simulink model "dron_filtro_complementario_version2015_Orientacion2"  (R2015b)
settings: Solver=FixedStepDiscrete  StartTime=0.0  StopTime=inf  FixedStep=0.03  RelTol=1e-3
undefined symbols (not defined in the file): DiscIntNeverNeededParam
libraries: simulink x5, arduinolib x4, RASPlib x2
settings Model: SimulationMode=external  ExtModeTrigDuration=2  Creator=jorge  LastModifiedBy=jorge
settings OptimizationCC: OptimizeModelRefInitCode=on  LifeSpan=Inf  MaxStackSize=64
settings HardwareCC: ProdBitPerInt=16  ProdBitPerPointer=16  ProdLargestAtomicFloat=None  ProdWordSize=8  ProdHWDeviceType=Atmel->AVR
settings RTWCC: SystemTargetFile=ert.tlc  TemplateMakefile=ert_default_tmf  Description=Embedded Coder  Toolchain=Arduino AVR v1.6.1  BuildConfiguration=Faster Runs
settings CodeAppCC: IgnoreCustomStorageClasses=off
settings ERTTargetCC: SupportContinuousTime=on  SupportVariableSizeSignals=on  ExtMode=on  ExtModeMexFile=ext_serial_win32_comm_rtt  ExtModeMexArgs=0 5 115200

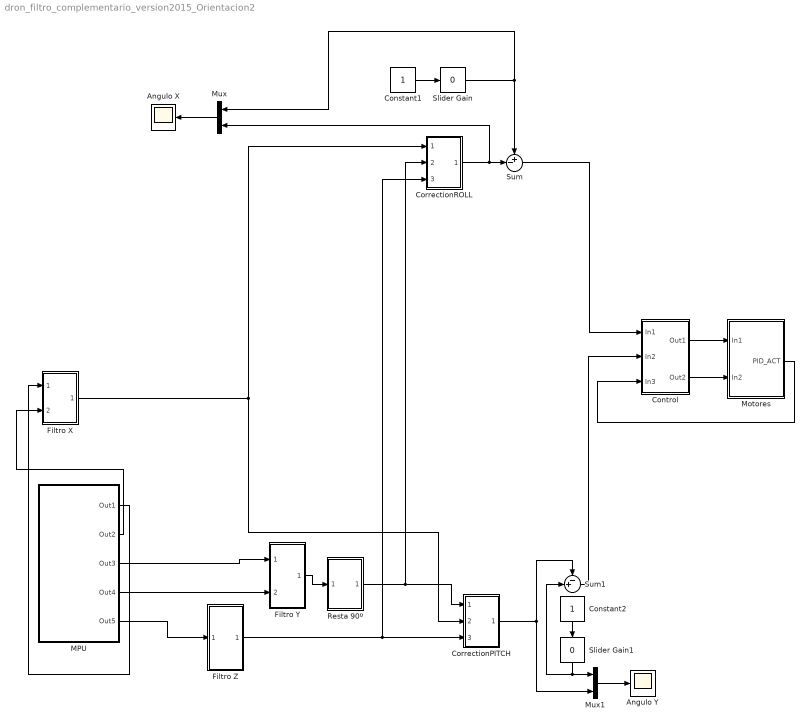
== system dron_filtro_complementario_version2015_Orientacion2 ==
  Angulo X : Scope
  Angulo Y : Scope
  Constant1 : Constant
  Constant2 : Constant
  Control : Subsystem
  CorrectionPITCH : Subsystem
  CorrectionROLL : Subsystem
  Filtro X : Subsystem
  Filtro Y : Subsystem
  "Filtro Z " : Subsystem
  "MPU " : Subsystem
  "Motores " : Subsystem
  Mux : Mux  Inputs=2
  Mux1 : Mux  Inputs=2
  Resta 90º : Subsystem
  Slider Gain : simulink/Math Operations/Slider Gain  low=-25  gain=0  high=35
  Slider Gain1 : simulink/Math Operations/Slider Gain  low=-25  gain=0  high=35
  Sum : Sum  Inputs=+-|
  Sum1 : Sum  Inputs=-+|
  wires:
  "MPU "/1(Out1) -> Filtro X/1(In1)
  "MPU "/2(Out2) -> Filtro X/2(In2)
  Mux/1 -> Angulo X/1
  Constant1/1 -> Slider Gain/1
  Slider Gain/1 -> Sum/1, Mux/1
  "MPU "/3(Out3) -> Filtro Y/1(In1)
  "MPU "/4(Out4) -> Filtro Y/2(In2)
  Constant2/1 -> Slider Gain1/1
  Mux1/1 -> Angulo Y/1
  "MPU "/5(Out5) -> "Filtro Z "/1(In1)
  Filtro X/1(Out3) -> CorrectionPITCH/2(In2), CorrectionROLL/1(In1)
  Slider Gain1/1 -> Mux1/1, Sum1/2
  Filtro Y/1(Out3) -> Resta 90º/1(In1)
  Resta 90º/1(Out1) -> CorrectionPITCH/1(In1), CorrectionROLL/2(In2)
  "Filtro Z "/1(Out3) -> CorrectionROLL/3(In3), CorrectionPITCH/3(In3)
  CorrectionPITCH/1(Out1) -> Sum1/1, Mux1/2
  CorrectionROLL/1(Out1) -> Sum/2, Mux/2
  Sum/1 -> Control/1(In1)
  Sum1/1 -> Control/2(In2)
  Control/1(Out1) -> "Motores "/1(In1)
  Control/2(Out2) -> "Motores "/2(In2)
  "Motores "/1("PID_ACT ") -> Control/3(In3)

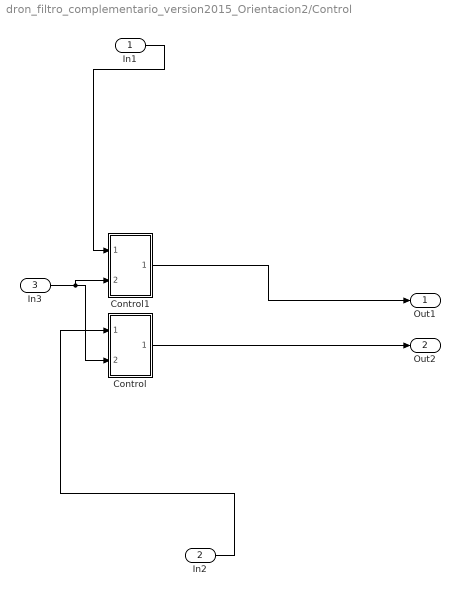
== system dron_filtro_complementario_version2015_Orientacion2/Control ==
  In1 : Inport
  In2 : Inport  Port=2
  In3 : Inport  Port=3
  Control : Subsystem
  Control1 : Subsystem
  Out1 : Outport
  Out2 : Outport  Port=2
  wires:
  Control1/1(Out1) -> Out1/1
  Control/1(Out1) -> Out2/1
  In2/1 -> Control/1(In1)
  In1/1 -> Control1/1(In1)
  In3/1 -> Control/2(Threshold), Control1/2(Threshold)

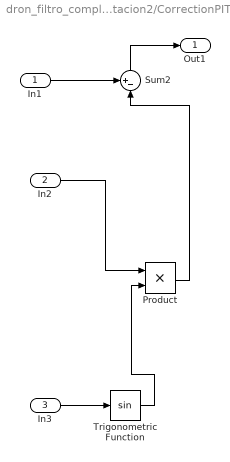
== system dron_filtro_complementario_version2015_Orientacion2/CorrectionPITCH ==
  In1 : Inport
  In2 : Inport  Port=2
  In3 : Inport  Port=3
  Product : Product
  Sum2 : Sum  Inputs=+-|
  Trigonometric Function : Trigonometry
  Out1 : Outport
  wires:
  Trigonometric Function/1 -> Product/2
  Product/1 -> Sum2/2
  In1/1 -> Sum2/1
  In3/1 -> Trigonometric Function/1
  Sum2/1 -> Out1/1
  In2/1 -> Product/1

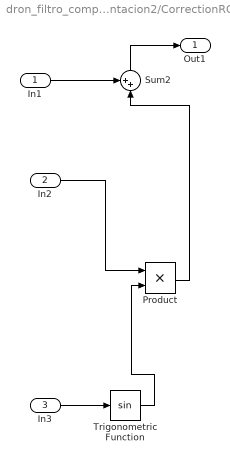
== system dron_filtro_complementario_version2015_Orientacion2/CorrectionROLL ==
  In1 : Inport
  In2 : Inport  Port=2
  In3 : Inport  Port=3
  Product : Product
  Sum2 : Sum  Inputs=++|
  Trigonometric Function : Trigonometry
  Out1 : Outport
  wires:
  Trigonometric Function/1 -> Product/2
  Product/1 -> Sum2/2
  In1/1 -> Sum2/1
  In3/1 -> Trigonometric Function/1
  Sum2/1 -> Out1/1
  In2/1 -> Product/1

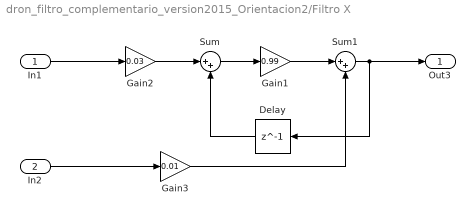
== system dron_filtro_complementario_version2015_Orientacion2/Filtro X ==
  In1 : Inport
  In2 : Inport  Port=2
  Delay : Delay  DelayLength=1  InitialCondition=0
  Gain1 : Gain  Gain=0.99
  Gain2 : Gain  Gain=0.03
  Gain3 : Gain  Gain=0.01
  Sum : Sum  Inputs=|++
  Sum1 : Sum  Inputs=|++
  Out3 : Outport
  wires:
  Delay/1 -> Sum/2
  Sum/1 -> Gain1/1
  In2/1 -> Gain3/1
  Gain1/1 -> Sum1/1
  Sum1/1 -> Out3/1, Delay/1
  In1/1 -> Gain2/1
  Gain2/1 -> Sum/1
  Gain3/1 -> Sum1/2

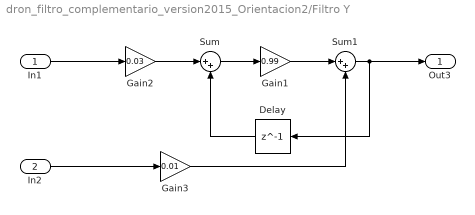
== system dron_filtro_complementario_version2015_Orientacion2/Filtro Y ==
  In1 : Inport
  In2 : Inport  Port=2
  Delay : Delay  DelayLength=1  InitialCondition=0
  Gain1 : Gain  Gain=0.99
  Gain2 : Gain  Gain=0.03
  Gain3 : Gain  Gain=0.01
  Sum : Sum  Inputs=|++
  Sum1 : Sum  Inputs=|++
  Out3 : Outport
  wires:
  Delay/1 -> Sum/2
  Sum/1 -> Gain1/1
  In2/1 -> Gain3/1
  Gain1/1 -> Sum1/1
  Sum1/1 -> Out3/1, Delay/1
  In1/1 -> Gain2/1
  Gain2/1 -> Sum/1
  Gain3/1 -> Sum1/2

== system dron_filtro_complementario_version2015_Orientacion2/Filtro Z  ==
  In1 : Inport
  Discrete-Time Integrator : DiscreteIntegrator  InitialConditionSetting=State (most efficient)  SampleTime=-1  ICPrevOutput=DiscIntNeverNeededParam  ICPrevScaledInput=DiscIntNeverNeededParam
  Gain : Gain  Gain=3.1416/180
  Out3 : Outport
  wires:
  In1/1 -> Discrete-Time Integrator/1
  Gain/1 -> Out3/1
  Discrete-Time Integrator/1 -> Gain/1

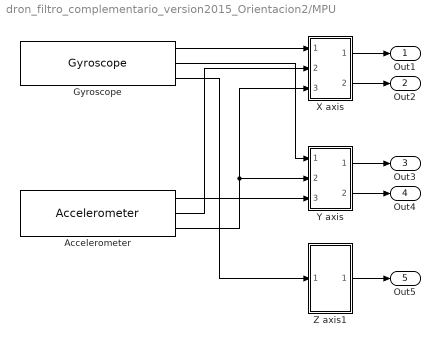
== system dron_filtro_complementario_version2015_Orientacion2/MPU  ==
  Accelerometer : RASPlib/Accelerometer  SimulateUsing=Code generation
  Gyroscope : RASPlib/Gyroscope  DLPFmode=0
  X axis : Subsystem
  Y axis : Subsystem
  Z axis1 : Subsystem
  Out1 : Outport
  Out2 : Outport  Port=2
  Out3 : Outport  Port=3
  Out4 : Outport  Port=4
  Out5 : Outport  Port=5
  wires:
  Gyroscope/3 -> Z axis1/1(In1)
  Gyroscope/1 -> X axis/1(In1)
  Accelerometer/2 -> X axis/2(In2)
  Accelerometer/3 -> Y axis/2(In2), X axis/3(In3)
  X axis/1(Out1) -> Out1/1
  X axis/2(Out2) -> Out2/1
  Gyroscope/2 -> Y axis/1(In1)
  Y axis/1(Out1) -> Out3/1
  Y axis/2(Out2) -> Out4/1
  Z axis1/1(Out1) -> Out5/1
  Accelerometer/1 -> Y axis/3(In3)

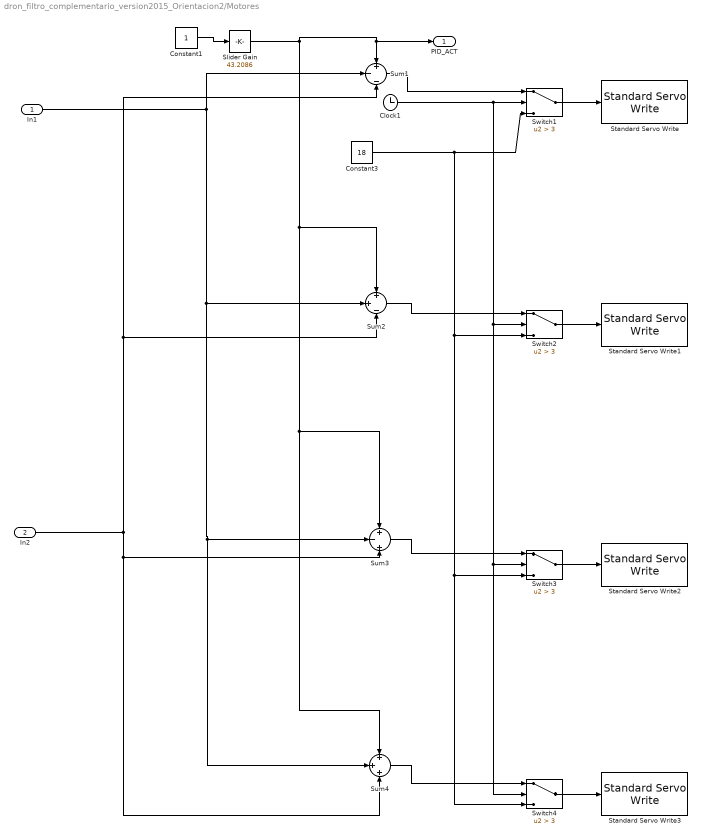
== system dron_filtro_complementario_version2015_Orientacion2/Motores  ==
  In1 : Inport
  In2 : Inport  Port=2
  Clock1 : Clock
  Constant1 : Constant
  Constant3 : Constant  Value=18
  Slider Gain : simulink/Math Operations/Slider Gain  low=0  gain=43.2086  high=60
  Standard Servo Write : arduinolib/Standard Servo Write  pinNumber=12  blockPlatform=arduino
  Standard Servo Write1 : arduinolib/Standard Servo Write  pinNumber=11  blockPlatform=arduino
  Standard Servo Write2 : arduinolib/Standard Servo Write  pinNumber=10  blockPlatform=arduino
  Standard Servo Write3 : arduinolib/Standard Servo Write  pinNumber=9  blockPlatform=arduino
  Sum1 : Sum  Inputs=+|-|-
  Sum2 : Sum  Inputs=+|+|-
  Sum3 : Sum  Inputs=+|-|+
  Sum4 : Sum  Inputs=+|+|+
  Switch{1..4} (4 alike) : Switch  Criteria=u2 > Threshold  Threshold=3
  "PID_ACT " : Outport
  wires:
  In2/1 -> Sum4/3, Sum3/3, Sum2/3, Sum1/3
  Constant3/1 -> Switch4/3, Switch3/3, Switch2/3, Switch1/3
  Slider Gain/1 -> "PID_ACT "/1, Sum1/1, Sum3/1, Sum4/1, Sum2/1
  Sum4/1 -> Switch4/1
  Clock1/1 -> Switch4/2, Switch3/2, Switch2/2, Switch1/2
  Sum3/1 -> Switch3/1
  Switch4/1 -> Standard Servo Write3/1
  Switch3/1 -> Standard Servo Write2/1
  Sum1/1 -> Switch1/1
  Switch1/1 -> Standard Servo Write/1
  Switch2/1 -> Standard Servo Write1/1
  Sum2/1 -> Switch2/1
  In1/1 -> Sum1/2, Sum4/2, Sum3/2, Sum2/2
  Constant1/1 -> Slider Gain/1

== system dron_filtro_complementario_version2015_Orientacion2/Resta 90º ==
  In1 : Inport
  Add : Sum  Inputs=+-
  resta90º : Constant  Value=90
  Out1 : Outport
  wires:
  resta90º/1 -> Add/2
  In1/1 -> Add/1
  Add/1 -> Out1/1

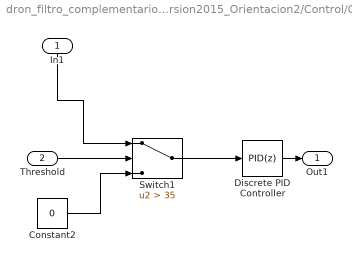
== system dron_filtro_complementario_version2015_Orientacion2/Control/Control ==
  In1 : Inport
  Threshold : Inport  Port=2
  Constant2 : Constant  Value=0
  Discrete PID Controller : simulink/Continuous/PID Controller  Controller=PID  TimeDomain=Discrete-time  SampleTime=-1  IntegratorMethod=Forward Euler  FilterMethod=Forward Euler  Form=Parallel  UseFilter=off  ControllerParametersSource=internal  P=0.51  I=0.425  D=0.106  N=30  InitialConditionSource=internal  InitialConditionForIntegrator=0  InitialConditionForFilter=0  ExternalReset=none  LimitOutput=off  UpperSaturationLimit=inf  LowerSaturationLimit=-inf  LinearizeAsGain=off  AntiWindupMode=none  Kb=1  TrackingMode=off  Kt=1  PParamMin=[]  PParamMax=[]  IParamMin=[]  IParamMax=[]  DParamMin=[]  DParamMax=[]  NParamMin=[]  NParamMax=[]  KbParamMin=[]  KbParamMax=[]  KtParamMin=[]  KtParamMax=[]  POutMin=[]  POutMax=[]  IOutMin=[]  IOutMax=[]  DOutMin=[]  DOutMax=[]  NOutMin=[]  NOutMax=[]  KbOutMin=[]  KbOutMax=[]  KtOutMin=[]  KtOutMax=[]  IntegratorOutMin=[]  IntegratorOutMax=[]  FilterOutMin=[]  FilterOutMax=[]  SumOutMin=[]  SumOutMax=[]  SumI1OutMin=[]  SumI1OutMax=[]  SumI2OutMin=[]  SumI2OutMax=[]  SumI3OutMin=[]  SumI3OutMax=[]  SumDOutMin=[]  SumDOutMax=[]  SaturationOutMin=[]  SaturationOutMax=[]  IntegratorContinuousStateAttributes=''  IntegratorStateMustResolveToSignalObject=off  IntegratorRTWStateStorageClass=Auto  FilterContinuousStateAttributes=''  FilterStateMustResolveToSignalObject=off  FilterRTWStateStorageClass=Auto  DifferentiatorICPrevScaledInput=0  DifferentiatorOutMin=[]  DifferentiatorOutMax=[]
  Switch1 : Switch  Criteria=u2 > Threshold  Threshold=35
  Out1 : Outport
  wires:
  Discrete PID Controller/1 -> Out1/1
  Switch1/1 -> Discrete PID Controller/1
  Threshold/1 -> Switch1/2
  Constant2/1 -> Switch1/3
  In1/1 -> Switch1/1

== system dron_filtro_complementario_version2015_Orientacion2/Control/Control1 ==
  In1 : Inport
  Threshold : Inport  Port=2
  Constant2 : Constant  Value=0
  Discrete PID Controller : simulink/Continuous/PID Controller  Controller=PID  TimeDomain=Discrete-time  SampleTime=-1  IntegratorMethod=Forward Euler  FilterMethod=Forward Euler  Form=Parallel  UseFilter=off  ControllerParametersSource=internal  P=0.51  I=0.425  D=0.106  N=30  InitialConditionSource=internal  InitialConditionForIntegrator=0  InitialConditionForFilter=0  ExternalReset=none  LimitOutput=off  UpperSaturationLimit=inf  LowerSaturationLimit=-inf  LinearizeAsGain=off  AntiWindupMode=none  Kb=1  TrackingMode=off  Kt=1  PParamMin=[]  PParamMax=[]  IParamMin=[]  IParamMax=[]  DParamMin=[]  DParamMax=[]  NParamMin=[]  NParamMax=[]  KbParamMin=[]  KbParamMax=[]  KtParamMin=[]  KtParamMax=[]  POutMin=[]  POutMax=[]  IOutMin=[]  IOutMax=[]  DOutMin=[]  DOutMax=[]  NOutMin=[]  NOutMax=[]  KbOutMin=[]  KbOutMax=[]  KtOutMin=[]  KtOutMax=[]  IntegratorOutMin=[]  IntegratorOutMax=[]  FilterOutMin=[]  FilterOutMax=[]  SumOutMin=[]  SumOutMax=[]  SumI1OutMin=[]  SumI1OutMax=[]  SumI2OutMin=[]  SumI2OutMax=[]  SumI3OutMin=[]  SumI3OutMax=[]  SumDOutMin=[]  SumDOutMax=[]  SaturationOutMin=[]  SaturationOutMax=[]  IntegratorContinuousStateAttributes=''  IntegratorStateMustResolveToSignalObject=off  IntegratorRTWStateStorageClass=Auto  FilterContinuousStateAttributes=''  FilterStateMustResolveToSignalObject=off  FilterRTWStateStorageClass=Auto  DifferentiatorICPrevScaledInput=0  DifferentiatorOutMin=[]  DifferentiatorOutMax=[]
  Switch1 : Switch  Criteria=u2 > Threshold  Threshold=35
  Out1 : Outport
  wires:
  Discrete PID Controller/1 -> Out1/1
  Switch1/1 -> Discrete PID Controller/1
  Threshold/1 -> Switch1/2
  Constant2/1 -> Switch1/3
  In1/1 -> Switch1/1

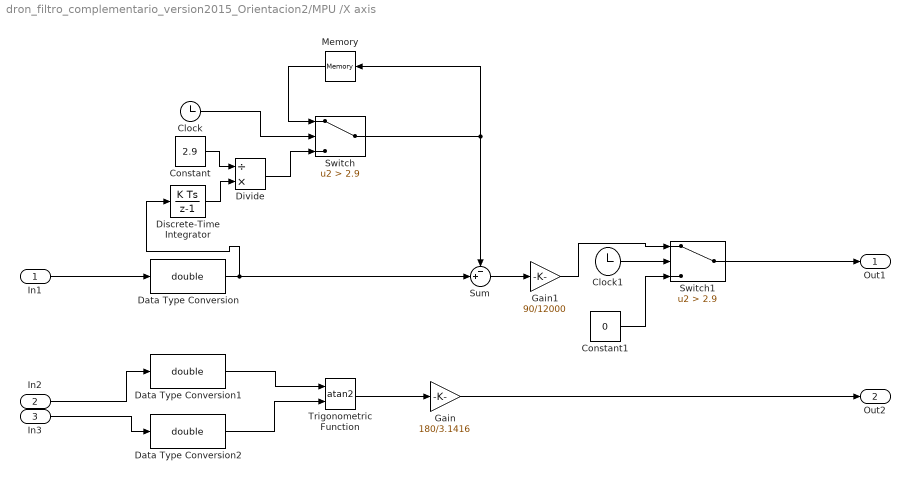
== system dron_filtro_complementario_version2015_Orientacion2/MPU /X axis ==
  In1 : Inport
  In2 : Inport  Port=2
  In3 : Inport  Port=3
  Clock : Clock
  Clock1 : Clock
  Constant : Constant  Value=2.9
  Constant1 : Constant  Value=0
  Data Type Conversion : DataTypeConversion  OutDataTypeStr=double
  Data Type Conversion1 : DataTypeConversion  OutDataTypeStr=double
  Data Type Conversion2 : DataTypeConversion  OutDataTypeStr=double
  Discrete-Time Integrator : DiscreteIntegrator  InitialConditionSetting=State (most efficient)  SampleTime=-1  ICPrevOutput=DiscIntNeverNeededParam  ICPrevScaledInput=DiscIntNeverNeededParam
  Divide : Product  Inputs=/*
  Gain : Gain  Gain=180/3.1416
  Gain1 : Gain  Gain=90/12000
  Memory : Memory
  Sum : Sum  Inputs=-+|
  Switch : Switch  Criteria=u2 > Threshold  Threshold=2.9
  Switch1 : Switch  Criteria=u2 > Threshold  Threshold=2.9
  Trigonometric Function : Trigonometry  Operator=atan2
  Out1 : Outport
  Out2 : Outport  Port=2
  wires:
  Sum/1 -> Gain1/1
  Clock/1 -> Switch/2
  Switch/1 -> Sum/1, Memory/1
  Constant/1 -> Divide/1
  Gain/1 -> Out2/1
  Clock1/1 -> Switch1/2
  Trigonometric Function/1 -> Gain/1
  Data Type Conversion/1 -> Sum/2, Discrete-Time Integrator/1
  Switch1/1 -> Out1/1
  Data Type Conversion1/1 -> Trigonometric Function/1
  Data Type Conversion2/1 -> Trigonometric Function/2
  In2/1 -> Data Type Conversion1/1
  Constant1/1 -> Switch1/3
  In3/1 -> Data Type Conversion2/1
  Divide/1 -> Switch/3
  Memory/1 -> Switch/1
  Discrete-Time Integrator/1 -> Divide/2
  In1/1 -> Data Type Conversion/1
  Gain1/1 -> Switch1/1

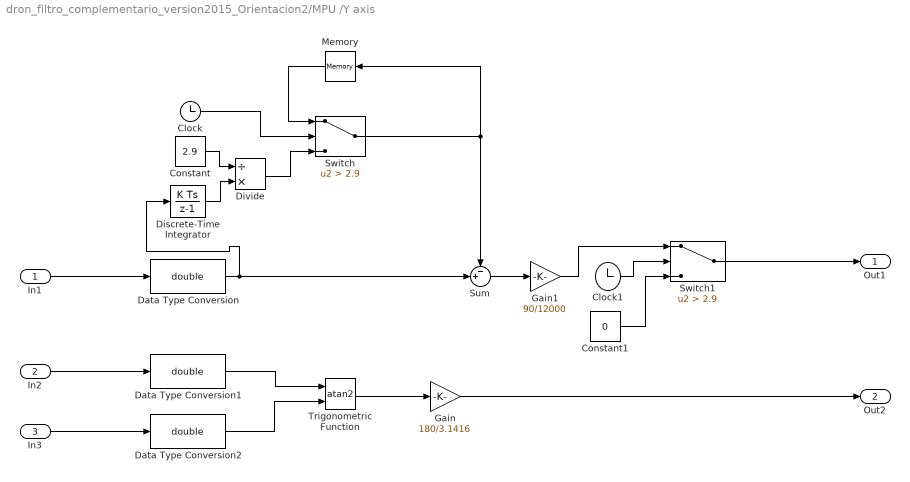
== system dron_filtro_complementario_version2015_Orientacion2/MPU /Y axis ==
  In1 : Inport
  In2 : Inport  Port=2
  In3 : Inport  Port=3
  Clock : Clock
  Clock1 : Clock
  Constant : Constant  Value=2.9
  Constant1 : Constant  Value=0
  Data Type Conversion : DataTypeConversion  OutDataTypeStr=double
  Data Type Conversion1 : DataTypeConversion  OutDataTypeStr=double
  Data Type Conversion2 : DataTypeConversion  OutDataTypeStr=double
  Discrete-Time Integrator : DiscreteIntegrator  InitialConditionSetting=State (most efficient)  SampleTime=-1  ICPrevOutput=DiscIntNeverNeededParam  ICPrevScaledInput=DiscIntNeverNeededParam
  Divide : Product  Inputs=/*
  Gain : Gain  Gain=180/3.1416
  Gain1 : Gain  Gain=90/12000
  Memory : Memory
  Sum : Sum  Inputs=-+|
  Switch : Switch  Criteria=u2 > Threshold  Threshold=2.9
  Switch1 : Switch  Criteria=u2 > Threshold  Threshold=2.9
  Trigonometric Function : Trigonometry  Operator=atan2
  Out1 : Outport
  Out2 : Outport  Port=2
  wires:
  Sum/1 -> Gain1/1
  Clock/1 -> Switch/2
  Switch/1 -> Sum/1, Memory/1
  Constant/1 -> Divide/1
  Gain/1 -> Out2/1
  Clock1/1 -> Switch1/2
  Trigonometric Function/1 -> Gain/1
  Data Type Conversion/1 -> Sum/2, Discrete-Time Integrator/1
  Switch1/1 -> Out1/1
  Data Type Conversion1/1 -> Trigonometric Function/1
  Data Type Conversion2/1 -> Trigonometric Function/2
  In2/1 -> Data Type Conversion1/1
  Constant1/1 -> Switch1/3
  In3/1 -> Data Type Conversion2/1
  Divide/1 -> Switch/3
  Memory/1 -> Switch/1
  Discrete-Time Integrator/1 -> Divide/2
  In1/1 -> Data Type Conversion/1
  Gain1/1 -> Switch1/1

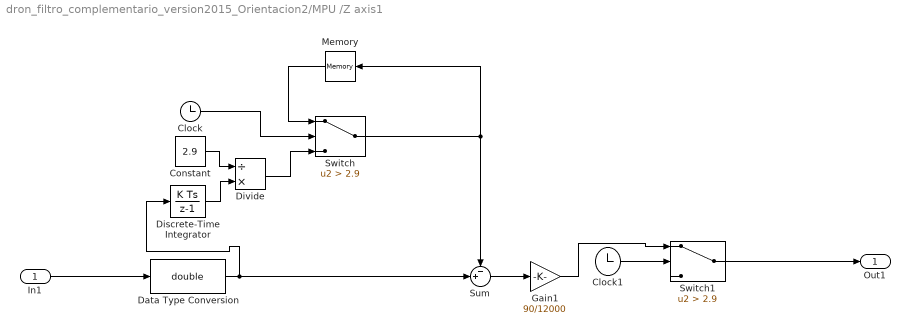
== system dron_filtro_complementario_version2015_Orientacion2/MPU /Z axis1 ==
  In1 : Inport
  Clock : Clock
  Clock1 : Clock
  Constant : Constant  Value=2.9
  Data Type Conversion : DataTypeConversion  OutDataTypeStr=double
  Discrete-Time Integrator : DiscreteIntegrator  InitialConditionSetting=State (most efficient)  SampleTime=-1  ICPrevOutput=DiscIntNeverNeededParam  ICPrevScaledInput=DiscIntNeverNeededParam
  Divide : Product  Inputs=/*
  Gain1 : Gain  Gain=90/12000
  Memory : Memory
  Sum : Sum  Inputs=-+|
  Switch : Switch  Criteria=u2 > Threshold  Threshold=2.9
  Switch1 : Switch  Criteria=u2 > Threshold  Threshold=2.9
  Out1 : Outport
  wires:
  Sum/1 -> Gain1/1
  Clock/1 -> Switch/2
  Switch/1 -> Sum/1, Memory/1
  Constant/1 -> Divide/1
  Clock1/1 -> Switch1/2
  Data Type Conversion/1 -> Sum/2, Discrete-Time Integrator/1
  Switch1/1 -> Out1/1
  ? -> Switch1/3
  Divide/1 -> Switch/3
  Memory/1 -> Switch/1
  Discrete-Time Integrator/1 -> Divide/2
  In1/1 -> Data Type Conversion/1
  Gain1/1 -> Switch1/1
